simulink model "flexible_joint_v2"  (R2023b)
settings: Solver=VariableStepAuto  StartTime=0.0  StopTime=40  RelTol=1e-3
libraries: simulink x2
settings Model: Creator=GreenTeam  LastModifiedBy=GreenTeam

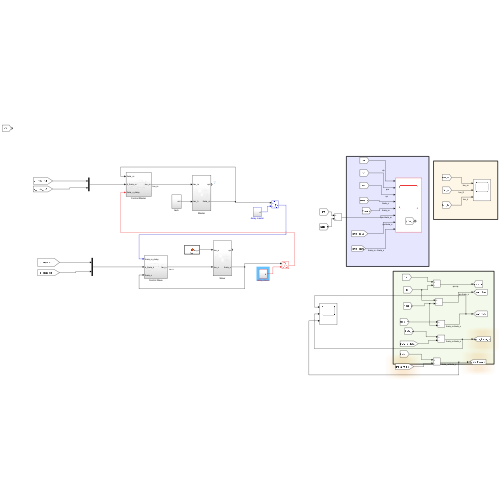
[thumbnail: Simulink's stored preview of the top-level diagram]
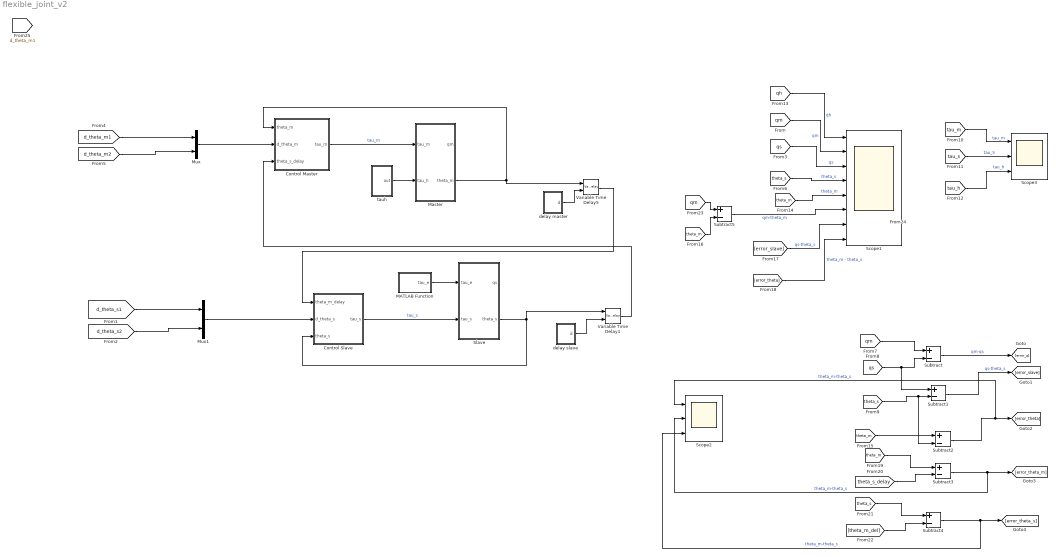
== system flexible_joint_v2 ==
  Control Master : Subsystem
  Control Slave : Subsystem
  MATLAB Function : MATLAB Function  TreatAsAtomicUnit=on
  Master : Subsystem
  Mux : Mux  Inputs=2
  Mux1 : Mux  Inputs=2
  Scope1 : Scope  NumInputPorts=8
  Scope2 : Scope  NumInputPorts=3
  Scope3 : Scope  NumInputPorts=3
  Slave : Subsystem
  Subtract{,1..5} (6 alike) : Sum  Inputs=+-
  Variable Time Delay1 : VariableTransportDelay  MaximumDelay=10  MaximumPoints=499712
  Variable Time Delay5 : VariableTransportDelay  MaximumDelay=10  MaximumPoints=499712
  delay master : Subsystem
  delay slave : Subsystem
  tauh : Subsystem
  wires:
  [tau_h] -> Scope3/3  "tau_h"
  [qm] -> Subtract/1
  [tau_s] -> Scope3/2  "tau_S"
  delay slave/1(d) -> Variable Time Delay1/2
  Subtract2/1 -> Scope2/1, [error_theta]  "theta_m-theta_s"
  [d_theta_m2] -> Mux/2
  Subtract1/1 -> [error_slave]  "qs-theta_s"
  Subtract/1 -> [error_q]  "qm-qs"
  [qs] -> Subtract1/1, Subtract/2
  delay master/1(d) -> Variable Time Delay5/2
  [d_theta_s2] -> Mux1/2
  Mux/1 -> Control Master/2(d_theta_m)
  [theta_s] -> Scope1/4  "theta_s"
  [qs] -> Scope1/3  "qs"
  [theta_s] -> Subtract2/2, Subtract1/2
  Mux1/1 -> Control Slave/2(d_theta_s)
  MATLAB Function/1(tau_e) -> Slave/1(tau_e)
  Slave/2(theta_s) -> Control Slave/3(theta_s), Variable Time Delay1/1
  [qm] -> Scope1/2  "qm"
  [d_theta_s1] -> Mux1/1
  [d_theta_m1] -> Mux/1
  Control Slave/1(tau_s) -> Slave/2(tau_s)  "tau_s"
  [qh] -> Scope1/1  "qh"
  Variable Time Delay5/1 -> Control Slave/1(theta_m_delay)
  [tau_m] -> Scope3/1  "tau_m"
  Variable Time Delay1/1 -> Control Master/3(theta_s_delay)
  Master/2(theta_m) -> Variable Time Delay5/1, Control Master/1(theta_m)
  [theta_m] -> Scope1/5  "theta_m"
  tauh/1(out) -> Master/2(tau_h)
  Control Master/1(tau_m) -> Master/1(tau_m)  "tau_m"
  [theta_m] -> Subtract2/1
  Subtract5/1 -> Scope1/6  "qm-theta_m"
  [error_slave] -> Scope1/7  "qs-theta_s"
  [error_theta] -> Scope1/8  "theta_m - theta_s"
  Subtract3/1 -> Scope2/2, [error_theta_m]  "theta_m-theta_s"
  [theta_m] -> Subtract3/1
  [theta_s_delay] -> Subtract3/2
  [theta_m_del] -> Subtract4/2
  [theta_s] -> Subtract4/1
  Subtract4/1 -> Scope2/3, [error_theta_s]  "theta_m-theta_s"
  [qm] -> Subtract5/1
  [theta_m] -> Subtract5/2

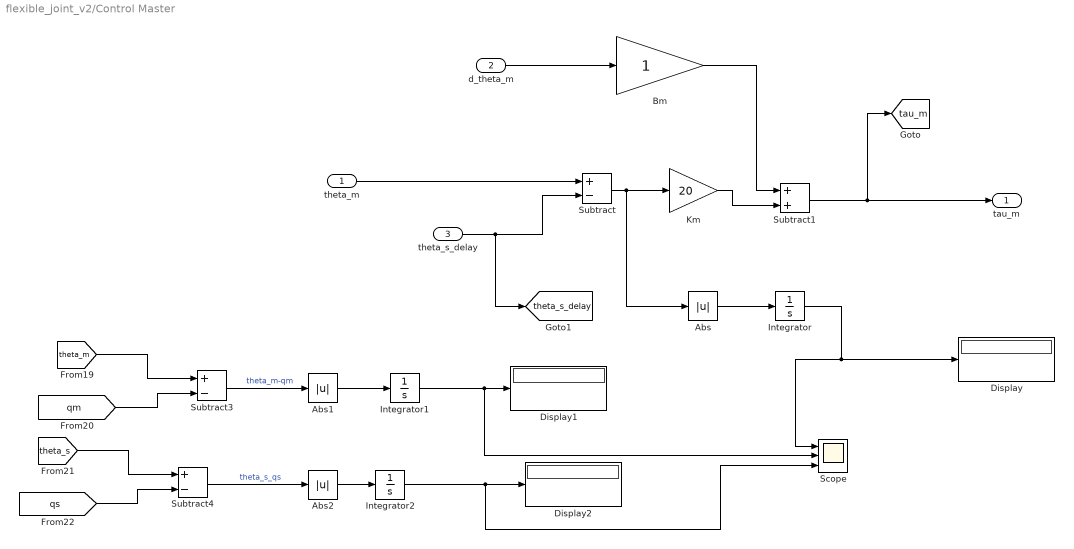
== system flexible_joint_v2/Control Master ==
  theta_m : Inport
  d_theta_m : Inport  Port=2
  theta_s_delay : Inport  Port=3
  Abs : Abs  SaturateOnIntegerOverflow=off
  Abs1 : Abs  SaturateOnIntegerOverflow=off
  Abs2 : Abs  SaturateOnIntegerOverflow=off
  Bm : Gain
  Display : Display
  Display1 : Display
  Display2 : Display
  Integrator : Integrator
  Integrator1 : Integrator
  Integrator2 : Integrator
  Km : Gain  Gain=20
  Scope : Scope  NumInputPorts=3
  Subtract : Sum  Inputs=+-
  Subtract1 : Sum
  Subtract3 : Sum  Inputs=+-
  Subtract4 : Sum  Inputs=+-
  tau_m : Outport
  tag scope: tau_m=global, theta_s_delay=global
  wires:
  Bm/1 -> Subtract1/1
  Subtract/1 -> Abs/1, Km/1
  Subtract1/1 -> [tau_m], tau_m/1
  Km/1 -> Subtract1/2
  d_theta_m/1 -> Bm/1
  theta_m/1 -> Subtract/1
  theta_s_delay/1 -> [theta_s_delay], Subtract/2
  Abs/1 -> Integrator/1
  Integrator/1 -> Display/1, Scope/1
  [theta_m] -> Subtract3/1
  [qm] -> Subtract3/2
  [theta_s] -> Subtract4/1
  [qs] -> Subtract4/2
  Subtract3/1 -> Abs1/1  "theta_m-qm"
  Subtract4/1 -> Abs2/1  "theta_s_qs"
  Abs1/1 -> Integrator1/1
  Abs2/1 -> Integrator2/1
  Integrator2/1 -> Scope/3, Display2/1
  Integrator1/1 -> Scope/2, Display1/1

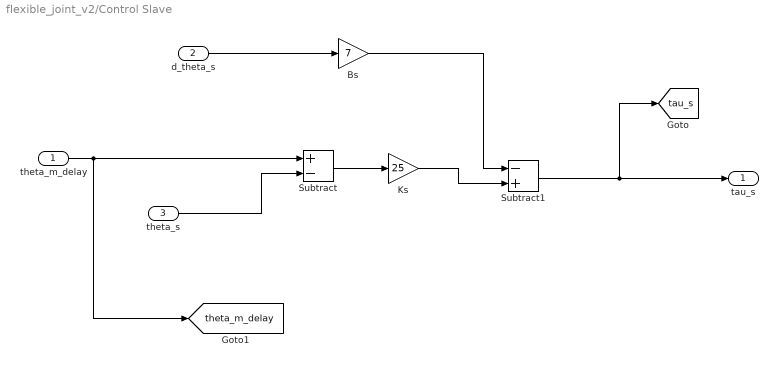
== system flexible_joint_v2/Control Slave ==
  theta_m_delay : Inport
  d_theta_s : Inport  Port=2
  theta_s : Inport  Port=3
  Bs : Gain  Gain=7
  Ks : Gain  Gain=25
  Subtract : Sum  Inputs=+-
  Subtract1 : Sum  Inputs=-+
  tau_s : Outport
  tag scope: tau_s=global, theta_m_delay=global
  wires:
  theta_s/1 -> Subtract/2
  theta_m_delay/1 -> [theta_m_delay], Subtract/1
  d_theta_s/1 -> Bs/1
  Ks/1 -> Subtract1/2
  Subtract1/1 -> [tau_s], tau_s/1
  Subtract/1 -> Ks/1
  Bs/1 -> Subtract1/1

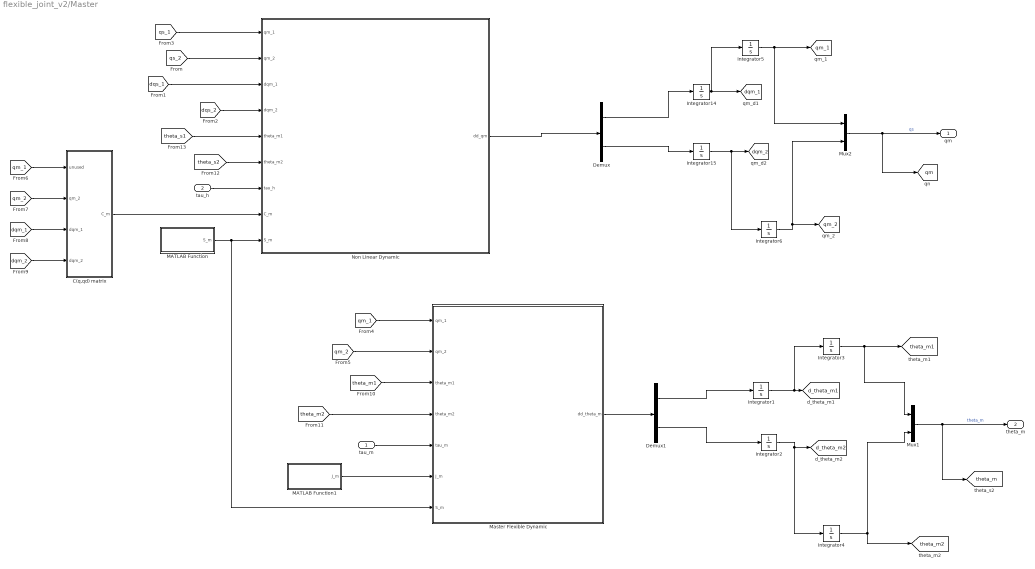
== system flexible_joint_v2/Master ==
  tau_m : Inport
  tau_h : Inport  Port=2
  C(q,qd) matrix : MATLAB Function  TreatAsAtomicUnit=on
  Demux : Demux  Outputs=2
  Demux1 : Demux  Outputs=2
  Integrator{1..4,14..15} (6 alike) : Integrator
  Integrator5 : Integrator  InitialCondition=-0.1
  Integrator6 : Integrator  InitialCondition=0.1
  MATLAB Function : MATLAB Function  TreatAsAtomicUnit=on
  MATLAB Function1 : MATLAB Function  TreatAsAtomicUnit=on
  Master Flexible Dynamic : MATLAB Function  TreatAsAtomicUnit=on
  Mux1 : Mux  Inputs=2
  Mux2 : Mux  Inputs=2
  Non Linear Dynamic : MATLAB Function  TreatAsAtomicUnit=on
  qm : Outport
  theta_m : Outport  Port=2
  tag scope: d_theta_m1=global, d_theta_m2=global, dqm_1=global, dqm_2=global, qm=global, qm_1=global, qm_2=global, theta_m1=global, theta_m2=global, theta_m=global
  wires:
  tau_m/1 -> Master Flexible Dynamic/5(tau_m)
  tau_h/1 -> Non Linear Dynamic/7(tau_h)
  [theta_s1] -> Non Linear Dynamic/5(theta_m1)
  [theta_s2] -> Non Linear Dynamic/6(theta_m2)
  [theta_m2] -> Master Flexible Dynamic/4(theta_m2)
  [theta_m1] -> Master Flexible Dynamic/3(theta_m1)
  [qm_2] -> Master Flexible Dynamic/2(qm_2)
  [qm_1] -> Master Flexible Dynamic/1(qm_1)
  Demux1/2 -> Integrator2/1
  Mux1/1 -> theta_m/1, [theta_m]  "theta_m"
  Integrator2/1 -> [d_theta_m2], Integrator4/1
  Integrator4/1 -> Mux1/2, [theta_m2]
  Master Flexible Dynamic/1(dd_theta_m) -> Demux1/1
  Demux1/1 -> Integrator1/1
  Integrator1/1 -> [d_theta_m1], Integrator3/1
  Integrator3/1 -> [theta_m1], Mux1/1
  MATLAB Function1/1(J_m) -> Master Flexible Dynamic/6(J_m)
  [qs_1] -> Non Linear Dynamic/1(qm_1)
  MATLAB Function/1(S_m) -> Master Flexible Dynamic/7(S_m), Non Linear Dynamic/9(S_m)
  C(q,qd) matrix/1(C_m) -> Non Linear Dynamic/8(C_m)
  Integrator5/1 -> [qm_1], Mux2/1
  Mux2/1 -> qm/1, [qm]  "qs"
  Demux/1 -> Integrator14/1
  Non Linear Dynamic/1(dd_qm) -> Demux/1
  Integrator6/1 -> [qm_2], Mux2/2
  Integrator14/1 -> Integrator5/1, [dqm_1]
  Integrator15/1 -> [dqm_2], Integrator6/1
  Demux/2 -> Integrator15/1
  [qs_2] -> Non Linear Dynamic/2(qm_2)
  [dqs_2] -> Non Linear Dynamic/4(dqm_2)
  [dqs_1] -> Non Linear Dynamic/3(dqm_1)
  [dqm_1] -> C(q,qd) matrix/3(dqm_1)
  [qm_1] -> C(q,qd) matrix/1(unused)
  [dqm_2] -> C(q,qd) matrix/4(dqm_2)
  [qm_2] -> C(q,qd) matrix/2(qm_2)

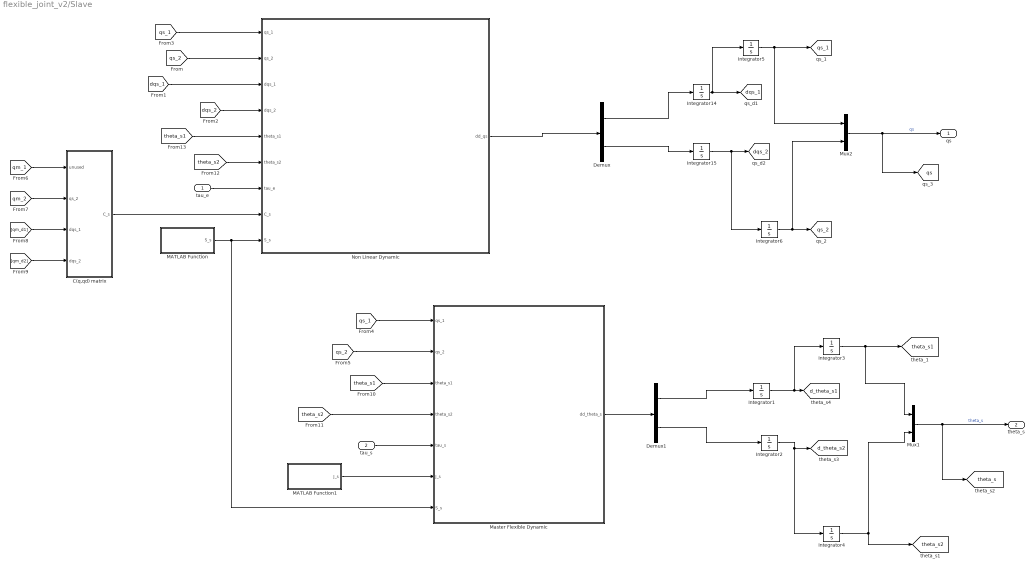
== system flexible_joint_v2/Slave ==
  tau_e : Inport
  tau_s : Inport  Port=2
  C(q,qd) matrix : MATLAB Function  TreatAsAtomicUnit=on
  Demux : Demux  Outputs=2
  Demux1 : Demux  Outputs=2
  Integrator{1..4,14..15} (6 alike) : Integrator
  Integrator5 : Integrator  InitialCondition=-0.1
  Integrator6 : Integrator  InitialCondition=0.1
  MATLAB Function : MATLAB Function  TreatAsAtomicUnit=on
  MATLAB Function1 : MATLAB Function  TreatAsAtomicUnit=on
  Master Flexible Dynamic : MATLAB Function  TreatAsAtomicUnit=on
  Mux1 : Mux  Inputs=2
  Mux2 : Mux  Inputs=2
  Non Linear Dynamic : MATLAB Function  TreatAsAtomicUnit=on
  qs : Outport
  theta_s : Outport  Port=2
  tag scope: d_theta_s1=global, d_theta_s2=global, dqs_1=global, dqs_2=global, qs=global, qs_1=global, qs_2=global, theta_s1=global, theta_s2=global, theta_s=global
  wires:
  [qm_2] -> C(q,qd) matrix/2(qs_2)
  [qm_d2] -> C(q,qd) matrix/4(dqs_2)
  [qm_1] -> C(q,qd) matrix/1(unused)
  [qm_d1] -> C(q,qd) matrix/3(dqs_1)
  [dqs_1] -> Non Linear Dynamic/3(dqs_1)
  [dqs_2] -> Non Linear Dynamic/4(dqs_2)
  [qs_2] -> Non Linear Dynamic/2(qs_2)
  Demux/2 -> Integrator15/1
  Integrator15/1 -> Integrator6/1, [dqs_2]
  Integrator14/1 -> [dqs_1], Integrator5/1
  Integrator6/1 -> Mux2/2, [qs_2]
  Non Linear Dynamic/1(dd_qs) -> Demux/1
  Demux/1 -> Integrator14/1
  Mux2/1 -> [qs], qs/1  "qs"
  Integrator5/1 -> Mux2/1, [qs_1]
  C(q,qd) matrix/1(C_s) -> Non Linear Dynamic/8(C_s)
  MATLAB Function/1(S_s) -> Non Linear Dynamic/9(S_s), Master Flexible Dynamic/7(S_s)
  [qs_1] -> Non Linear Dynamic/1(qs_1)
  MATLAB Function1/1(J_s) -> Master Flexible Dynamic/6(J_s)
  Integrator3/1 -> Mux1/1, [theta_s1]
  Integrator1/1 -> Integrator3/1, [d_theta_s1]
  Demux1/1 -> Integrator1/1
  Master Flexible Dynamic/1(dd_theta_s) -> Demux1/1
  Integrator4/1 -> [theta_s2], Mux1/2
  Integrator2/1 -> Integrator4/1, [d_theta_s2]
  Mux1/1 -> [theta_s], theta_s/1  "theta_s"
  Demux1/2 -> Integrator2/1
  [qs_1] -> Master Flexible Dynamic/1(qs_1)
  [qs_2] -> Master Flexible Dynamic/2(qs_2)
  [theta_s1] -> Master Flexible Dynamic/3(theta_s1)
  [theta_s2] -> Master Flexible Dynamic/4(theta_s2)
  [theta_s2] -> Non Linear Dynamic/6(theta_s2)
  [theta_s1] -> Non Linear Dynamic/5(theta_s1)
  tau_e/1 -> Non Linear Dynamic/7(tau_e)
  tau_s/1 -> Master Flexible Dynamic/5(tau_s)

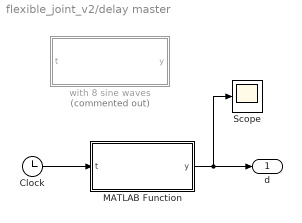
== system flexible_joint_v2/delay master ==
  Clock : Clock
  MATLAB Function : MATLAB Function  TreatAsAtomicUnit=on
  Scope : Scope
  with 8 sine waves : MATLAB Function  Commented=on  TreatAsAtomicUnit=on
  d : Outport
  wires:
  MATLAB Function/1(y) -> Scope/1, d/1
  Clock/1 -> MATLAB Function/1(t)

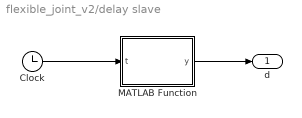
== system flexible_joint_v2/delay slave ==
  Clock : Clock
  MATLAB Function : MATLAB Function  TreatAsAtomicUnit=on
  d : Outport
  wires:
  Clock/1 -> MATLAB Function/1(t)
  MATLAB Function/1(y) -> d/1

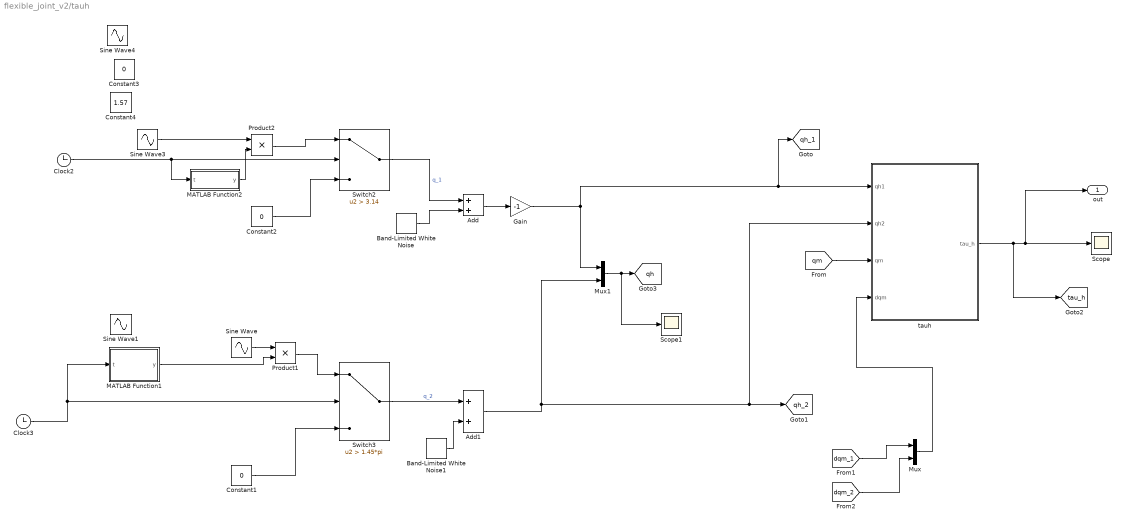
== system flexible_joint_v2/tauh ==
  Add : Sum
  Add1 : Sum
  Band-Limited White Noise : simulink/Sources/Band-Limited White Noise  Cov=[0.0001]  Ts=0.1  seed=[23341]
  Band-Limited White Noise1 : simulink/Sources/Band-Limited White Noise  Cov=[0.0001]  Ts=0.1  seed=[23341]
  Clock2 : Clock
  Clock3 : Clock
  Constant1 : Constant  Value=0
  Constant2 : Constant  Value=0
  Constant3 : Constant  Value=0
  Constant4 : Constant  Value=1.57
  Gain : Gain  Gain=-1
  MATLAB Function1 : MATLAB Function  TreatAsAtomicUnit=on
  MATLAB Function2 : MATLAB Function  TreatAsAtomicUnit=on
  Mux : Mux  Inputs=2
  Mux1 : Mux  Inputs=2
  Product1 : Product
  Product2 : Product
  Scope : Scope
  Scope1 : Scope
  Sine Wave : Sin  Amplitude=2.5  Frequency=1.5  SampleTime=0
  Sine Wave1 : Sin  Amplitude=0.2  Frequency=0.7  SampleTime=0
  Sine Wave3 : Sin  Amplitude=3  SampleTime=0
  Sine Wave4 : Sin  Amplitude=0.3  SampleTime=0
  Switch2 : Switch  Criteria=u2 > Threshold  Threshold=3.14  SaturateOnIntegerOverflow=off  InputSameDT=off
  Switch3 : Switch  Criteria=u2 > Threshold  Threshold=1.45*pi  SaturateOnIntegerOverflow=off  InputSameDT=off
  tauh : MATLAB Function  TreatAsAtomicUnit=on
  out : Outport
  tag scope: qh=global, qh_1=global, qh_2=global, tau_h=global
  wires:
  tauh/1(tau_h) -> [tau_h], out/1, Scope/1
  [dqm_1] -> Mux/1
  [dqm_2] -> Mux/2
  Mux/1 -> tauh/4(dqm)
  [qm] -> tauh/3(qm)
  Mux1/1 -> Scope1/1, [qh]
  Clock3/1 -> Switch3/2, MATLAB Function1/1(t)
  Clock2/1 -> MATLAB Function2/1(t), Switch2/2
  Switch2/1 -> Add/1  "q_1"
  Constant2/1 -> Switch2/3
  Add/1 -> Gain/1
  Band-Limited White Noise/1 -> Add/2
  MATLAB Function1/1(y) -> Product1/2
  Sine Wave/1 -> Product1/1
  Band-Limited White Noise1/1 -> Add1/2
  Switch3/1 -> Add1/1  "q_2"
  Add1/1 -> tauh/2(qh2), [qh_2], Mux1/2
  Gain/1 -> [qh_1], tauh/1(qh1), Mux1/1
  Sine Wave3/1 -> Product2/1
  MATLAB Function2/1(y) -> Product2/2
  Product2/1 -> Switch2/1
  Product1/1 -> Switch3/1
  Constant1/1 -> Switch3/3

== matlab function flexible_joint_v2/delay master/with 8 sine waves ==
  data: t input; y output
function y = reconstructed_signal(t)
    % Given data
    DC_offset = 0.9613888244716796;
    sine_amplitudes = [-0.02002779, -0.02351674, 0.00074362, 0.00154452, 0.0013555, -0.00135695, -0.00015931, 0.00089033];
    cosine_amplitudes = [-0.02562599, 0.00393932, -0.00523797, 0.0022634, 0.00295895, 0.00158273, -0.00018019, -0.0003756];
    frequencies = [0.24299065416927243, 0.48598130833854486, 0.7289719625078173, 0.9719626166770897, 1.2149532708463622, 1.4579439250156345, 1.7009345791849069, 1.9439252333541794];
    
    % Number of terms
    N = length(sine_amplitudes);
    
    % Initialize the signal
    y = DC_offset * ones(size(t));
    
    % Add sine and cosine terms
    for k = 1:N
        y = y + sine_amplitudes(k) * sin(2 * pi * frequencies(k) * t) + cosine_amplitudes(k) * cos(2 * pi * frequencies(k) * t);
    end
end

== matlab function flexible_joint_v2/Master/MATLAB Function1 ==
  data: J_m output
function J_m = Inertia_Matrix()

    % Create a 2x2 identity matrix
    I = eye(2);
    % Scale the identity matrix by 500
    J_m = 0.3 * I;
end

== matlab function flexible_joint_v2/Master/Master Flexible Dynamic ==
  data: qm_1 input; qm_2 input; theta_m1 input; dd_theta_m output; theta_m2 input; tau_m input; J_m input; S_m input
function dd_theta_m = Flex_Body_Master(qm_1,qm_2,theta_m1,theta_m2,tau_m,J_m,S_m)

q_m=[qm_1;qm_2];
theta_m=[theta_m1;theta_m2];


dd_theta_m = inv(J_m)*(-tau_m - S_m*(theta_m-q_m));

end

== matlab function flexible_joint_v2/Master/Non Linear Dynamic ==
  data: qm_1 input; qm_2 input; dqm_1 input; dqm_2 input; theta_m1 input; theta_m2 input; dd_qm output; tau_h input; C_m input; S_m input
function dd_qm =Rigid_Body_Master(qm_1,qm_2,dqm_1,dqm_2,theta_m1,theta_m2,tau_h,C_m,S_m)

% Phyiscal Parameters
Lm1 = 0.38;                                          %Master_first_link_length
Lm2 = 0.38;                                          %Master_second_link_length
mm1 = 3.947368;                                           %Master_first_link_mass
mm2 = 0.62326;                                           %Master_second_link_mass

qm=[qm_1;qm_2];
theta_m=[theta_m1;theta_m2];
dqm=[dqm_1;dqm_2];
alpha_m=(Lm2^2)*mm2+(Lm1^2)*(mm1+mm2);
betha_m=Lm1*Lm2*mm2;
delta_m=(Lm2^2)*mm2;

M_m_11= alpha_m + 2*betha_m*cos(qm_2);  
M_m_12= delta_m + betha_m * cos(qm_2);
M_m_21= M_m_12;
M_m_22= delta_m;
M_m = [M_m_11 M_m_12; M_m_21 M_m_22];
dd_qm= inv(M_m)*(tau_h  - (C_m * dqm ) - (S_m*(qm-theta_m)));
end

== matlab function flexible_joint_v2/tauh/MATLAB Function2 ==
  data: t input; y output
function y = exp_decay(t)
alpha=0.1;
y = exp(-alpha*t);

== matlab function flexible_joint_v2/tauh/MATLAB Function1 ==
  data: t input; y output
function y = exp_decay(t)
alpha=0.1;
y = exp(-alpha*t);

== matlab function flexible_joint_v2/tauh/tauh ==
  data: qh1 input; qh2 input; qm input; tau_h output; dqm input
function tau_h = spring_damper(qh1,qh2,qm,dqm)

Kh=10;
Dh=2;

qh=[qh1;qh2];
tau_h=Kh*(qh-qm)-Dh*dqm;


end

== matlab function flexible_joint_v2/Master/C(q,qd) matrix ==
  data: unused input; qm_2 input; dqm_1 input; C_m output; dqm_2 input
function C_m = fcn(~,qm_2,dqm_1,dqm_2)

% Phyiscal Parameters
Lm1 = 0.38;                                          %Master_first_link_length
Lm2 = 0.38;                                          %Master_second_link_length
mm1 = 3.947368;                                           %Master_first_link_mass
mm2 = 0.62326;                                           %Master_second_link_mass

betha_m=Lm1*Lm2*mm2;

C_m_11 = -1*betha_m*sin(qm_2)*dqm_2;
C_m_12 = -betha_m*sin(qm_2)*(dqm_1+dqm_2);
C_m_21 =  betha_m*sin(qm_2)*dqm_1;
C_m_22 =  0;
C_m = [C_m_11 C_m_12; C_m_21 C_m_22];
end

== matlab function flexible_joint_v2/delay master/MATLAB Function ==
  data: t input; y output
function y = reconstructed_signal(t)
    % Given data
    DC_offset = 0.9613462407597305;
    sine_amplitudes = [-0.02000659, -0.02349457, 0.00067474, 0.00159032, 0.00129016, -0.00135477, -0.00022001, 0.00097632, 0.00021585, 0.00014519, -0.00020833, -0.00056968, -0.00031181, 0.00016964, 0.0003376, -0.00022124];
    cosine_amplitudes = [-0.02556397, 0.00393168, -0.0052079, 0.00220769, 0.00300956, 0.00160663, -0.00018929, -0.00031848, -0.00019025, -0.00022222, -0.00010147, 0.00019351, -0.00030343, 0.0001225, 0.00015061, 0.00039704];
    frequencies = [0.24299065416927243, 0.48598130833854486, 0.7289719625078173, 0.9719626166770897, 1.2149532708463622, 1.4579439250156345, 1.7009345791849069, 1.9439252333541794, 2.186915887523452, 2.4299065416927244, 2.6728971958619967, 2.915887850031269, 3.1588785042005414, 3.4018691583698137, 3.6448598125390865, 3.887850466708359];
    
    % Number of terms
    N = length(sine_amplitudes);
    
    % Initialize the signal
    y = DC_offset * ones(size(t));
    
    % Add sine and cosine terms
    for k = 1:N
        y = y + sine_amplitudes(k) * sin(2 * pi * frequencies(k) * t) + cosine_amplitudes(k) * cos(2 * pi * frequencies(k) * t);
    end
    % dealy free
    %y=0;
end

== matlab function flexible_joint_v2/Master/MATLAB Function ==
  data: S_m output
function S_m = Stifness_Matrix()
    % This function creates a 2x2 identity matrix scaled by 500

    % Create a 2x2 identity matrix
    I = eye(2);
    
    % Scale the identity matrix by 500
    S_m = 100 * I;
end

== matlab function flexible_joint_v2/Slave/C(q,qd) matrix ==
  data: unused input; qs_2 input; dqs_1 input; C_s output; dqs_2 input
function C_s = fcn(~,qs_2,dqs_1,dqs_2)

% Phyiscal Parameters
Ls1 = 0.38;                                          %Slave_first_link_length
Ls2 = 0.38;                                          %Slave_second_link_length
ms1 = 0.5;                                           %Slave_first_link_mass
ms2 = 0.35;                                          %Slave_second_link_mass

betha_s=Ls1*Ls2*ms2;

C_s_11 = -1*betha_s*sin(qs_2)*dqs_2;
C_s_12 = -1*betha_s*sin(qs_2)*(dqs_1+dqs_2);
C_s_21 =  betha_s*sin(qs_2)*dqs_1;
C_s_22 =  0;
C_s= [C_s_11 C_s_12; C_s_21 C_s_22];
end

== matlab function flexible_joint_v2/Slave/MATLAB Function ==
  data: S_s output
function S_s = Stifness_Matrix()
    % This function creates a 2x2 identity matrix scaled by 500

    % Create a 2x2 identity matrix
    I = eye(2);
    
    % Scale the identity matrix by 500
    S_s = 100 * I;
end

== matlab function flexible_joint_v2/Slave/Master Flexible Dynamic ==
  data: qs_1 input; qs_2 input; theta_s1 input; dd_theta_s output; theta_s2 input; tau_s input; J_s input; S_s input
function dd_theta_s = Flex_Body_Slave(qs_1,qs_2,theta_s1,theta_s2,tau_s,J_s,S_s)

qs=[qs_1;qs_2];
theta_s=[theta_s1;theta_s2];


dd_theta_s = inv(J_s)*(tau_s - S_s*(theta_s-qs));

end

== matlab function flexible_joint_v2/Slave/MATLAB Function1 ==
  data: J_s output
function J_s = Inertia_Matrix()

    % Create a 2x2 identity matrix
    I = eye(2);
    % Scale the identity matrix by 500
    J_s = 0.3 * I;
end

== matlab function flexible_joint_v2/MATLAB Function ==
  data: tau_e output
function tau_e = fcn()

tau_e=[0;0];

== matlab function flexible_joint_v2/Slave/Non Linear Dynamic ==
  data: qs_1 input; qs_2 input; dqs_1 input; dqs_2 input; theta_s1 input; theta_s2 input; dd_qs output; tau_e input; C_s input; S_s input
function dd_qs =Rigid_Body_Slave(qs_1,qs_2,dqs_1,dqs_2,theta_s1,theta_s2,tau_e,C_s,S_s)

% Phyiscal Parameters
Ls1 = 0.38;                                          %Slave_first_link_length
Ls2 = 0.38;                                          %Slave_second_link_length
ms1 = 0.5;                                           %Slave_first_link_mass
ms2 = 0.35;                                          %Slave_second_link_mass

qs=[qs_1;qs_2];
theta_s=[theta_s1;theta_s2];
dqs=[dqs_1;dqs_2];
alpha_s=(Ls2^2)*ms2+(Ls1^2)*(ms1+ms2);
betha_s=Ls1*Ls2*ms2;
delta_s=(Ls2^2)*ms2;

M_s_11= alpha_s + 2*betha_s*cos(qs_2);  
M_s_12= delta_s + betha_s * cos(qs_2);
M_s_21= M_s_12;
M_s_22= delta_s;
M_s = [M_s_11 M_s_12; M_s_21 M_s_22];
dd_qs= inv(M_s)*(- tau_e  - (C_s * dqs ) - (S_s*(qs-theta_s)));
end

== matlab function flexible_joint_v2/delay slave/MATLAB Function ==
  data: t input; y output
function y = reconstructed_signal(t)
    % Given data
    DC_offset = 0.9613462407597305;
    sine_amplitudes = [-0.02000659, -0.02349457, 0.00067474, 0.00159032, 0.00129016, -0.00135477, -0.00022001, 0.00097632, 0.00021585, 0.00014519, -0.00020833, -0.00056968, -0.00031181, 0.00016964, 0.0003376, -0.00022124];
    cosine_amplitudes = [-0.02556397, 0.00393168, -0.0052079, 0.00220769, 0.00300956, 0.00160663, -0.00018929, -0.00031848, -0.00019025, -0.00022222, -0.00010147, 0.00019351, -0.00030343, 0.0001225, 0.00015061, 0.00039704];
    frequencies = [0.24299065416927243, 0.48598130833854486, 0.7289719625078173, 0.9719626166770897, 1.2149532708463622, 1.4579439250156345, 1.7009345791849069, 1.9439252333541794, 2.186915887523452, 2.4299065416927244, 2.6728971958619967, 2.915887850031269, 3.1588785042005414, 3.4018691583698137, 3.6448598125390865, 3.887850466708359];
    
    % Number of terms
    N = length(sine_amplitudes);
    
    % Initialize the signal
    y = DC_offset * ones(size(t));
    
    % Add sine and cosine terms
    for k = 1:N
        y = y + sine_amplitudes(k) * sin(2 * pi * frequencies(k) * t) + cosine_amplitudes(k) * cos(2 * pi * frequencies(k) * t);
    end
    %delay free
    %y=0;
end
